simulink model "Tut_Week_8_timeDelay"  (R2016a)
settings: Solver=FixedStepAuto  StartTime=0.0  StopTime=10.0  FixedStep=0.01  RelTol=1e-3
values from neighbouring files (symbols this model uses):
  tau1 = 0.1    [Tut_week_8.m]
  tau2 = 0.2    [Tut_week_8.m]
  tau3 = 0.3    [Tut_week_8.m]
  tau4 = 0.45    [Tut_week_8.m]
settings Model: Creator=김태욱  LastModifiedBy=김태욱

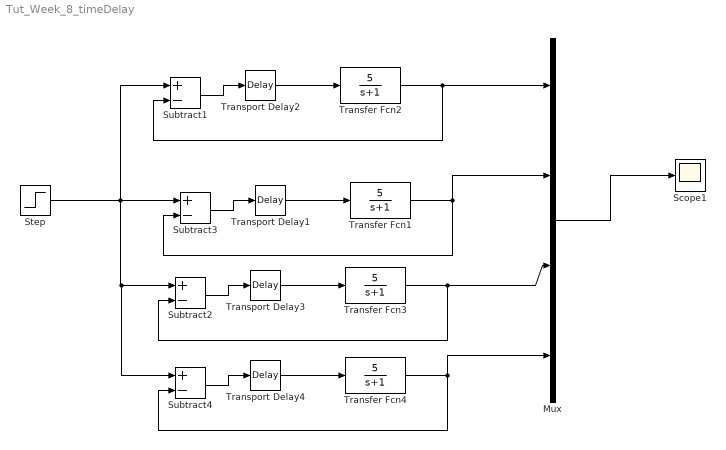
== system Tut_Week_8_timeDelay ==
  Mux : Mux
  Scope1 : Scope
  Step : Step  SampleTime=0
  Subtract{1..4} (4 alike) : Sum  Inputs=+-
  Transfer Fcn{1..4} (4 alike) : TransferFcn  Numerator=[5]  Denominator=[1 1]
  Transport Delay1 : TransportDelay  DelayTime=tau2
  Transport Delay2 : TransportDelay  DelayTime=tau1
  Transport Delay3 : TransportDelay  DelayTime=tau3
  Transport Delay4 : TransportDelay  DelayTime=tau4
  wires:
  Subtract3/1 -> Transport Delay1/1
  Transport Delay1/1 -> Transfer Fcn1/1
  Transfer Fcn1/1 -> Subtract3/2, Mux/2
  Subtract1/1 -> Transport Delay2/1
  Transport Delay2/1 -> Transfer Fcn2/1
  Transfer Fcn2/1 -> Mux/1, Subtract1/2
  Mux/1 -> Scope1/1
  Subtract2/1 -> Transport Delay3/1
  Transport Delay3/1 -> Transfer Fcn3/1
  Transfer Fcn3/1 -> Mux/3, Subtract2/2
  Step/1 -> Subtract4/1, Subtract2/1, Subtract1/1, Subtract3/1
  Subtract4/1 -> Transport Delay4/1
  Transport Delay4/1 -> Transfer Fcn4/1
  Transfer Fcn4/1 -> Subtract4/2, Mux/4
